simulink library "tqd"  (R2021b)
settings: Solver=VariableStepAuto  StartTime=0.0  StopTime=10.0  RelTol=1e-3
undefined symbols (not defined in the file): ATQD_AfterTqMinGain_X_Deg, ATQD_APSCreepBaseTqD_X_kph, ATQD_APSCreepBaseTqD_Y_Deg, ATQD_APSCreepBaseTqR_X_kph, ATQD_APSCreepBaseTqR_Y_Deg, ATQD_APSCreepIterm_X_kph, ATQD_APSCreepIterm_Y_kph, ATQD_APSCreepPterm_X_kph, ATQD_APSCreepPterm_Y_kph, ATQD_APSDecReq_X_kph, ATQD_APSDecReq_Y_mps2, ATQD_APSDecReqCMD_X_kph, ATQD_APSDecReqTs_X_pct, ATQD_APSDecTimeGain_X_Deg, ATQD_APSDecTimeGain_Y_s, ATQD_APSReqLowSpd_X_Deg, ATQD_AutoHoldReleaseBPS_X_Deg, ATQD_AWDLoadTrqnsGain_X_kg, ATQD_AWDLoadTrqnsGain_Y_pct, ATQD_BOSEnBPSPosn_X_kph, ATQD_BOSMap_X_rpm, ATQD_BOSMap_Y_pct, ATQD_CreepBaseTqD_X_kph, ATQD_CreepBaseTqD_Y_Deg, ATQD_CreepBaseTqR_X_kph, ATQD_CreepBaseTqR_Y_Deg, ATQD_CreepBPSDisPosn_X_Deg, ATQD_CreepBPSDisPosnR_X_Deg, ATQD_CreepBPSEnPosn_X_Deg, ATQD_CreepBPSEnPosnR_X_Deg, ATQD_CreepDeltaTq_X_kph, ATQD_CreepIterm_X_kph, ATQD_CreepIterm_Y_kph, ATQD_CreepItermMaxLimit_X_pct, ATQD_CreepPreloadTime_X_kph, ATQD_CreepPreloadTq_X_kph, ATQD_CreepPreloadTq_Y_s, ATQD_CreepProtTq_X_Deg, ATQD_CreepPterm_X_kph, ATQD_CreepPterm_Y_kph, ATQD_CreepRrTqSpRat_X_rpm, ATQD_CreepRrTqSpRat_Y_Nm, ATQD_CreepTargetSpdD_X_pct, ATQD_CreepTargetSpdR_X_pct, ATQD_ECOTqMapD_X_rpm, ATQD_ECOTqMapD_Y_pct, ATQD_EMTqMapD_X_rpm, ATQD_EMTqMapD_Y_pct, ATQD_EOPDTqMapDCon_X_rpm, ATQD_EOPDTqMapDCon_Y_Deg, ATQD_EscapeModePedTq_X_pct, ATQD_EscapeModePedTq_Y_rpm, ATQD_EscapeModePedTqFr_X_pct, ATQD_EscapeModePedTqFr_Y_rpm, ATQD_EstInitVehWeight_X_c, ATQD_FAfterTqCMDGain_X_rpm, ATQD_FAfterTqCMDGain_Y_pct, ATQD_FrLossMAPLowV_X_rpm, ATQD_FrLossMAPLowV_Y_Nm, ATQD_FrMotActReduce_X_rpm ... (+772)
libraries: simulink x211, hcu_lib x179, tqr x3
(part 10 of 28)

== system tqd/TQD/TorqueDemand/TorqueModule/OPD Hold ==
  task_time_s : Inport
  VTQD_RegenMode_enum : Inport  Port=2
  VTQD_GearActualPosn_enum : Inport  Port=3
  VTQD_VehActSpd_kph : Inport  Port=4
  VTQD_ActBPSPosn_pct : Inport  Port=5
  VVMC_ADASActive_flg : Inport  Port=6
  VVMC_CruzActive_flg : Inport  Port=7
  VTQD_ParkRequest_flg : Inport  Port=8
  VVMC_EstSlope_Deg : Inport  Port=9
  VVMC_LongAcc_Gps : Inport  Port=10
  VTQR_NoABSFEDUWhlTqReq_Nm : Inport  Port=11
  VTQR_NoABSREDUWhlTqReq_Nm : Inport  Port=12
  VINP_EPBSta_enum : Inport  Port=13
  VPMM_PwrSta_enum : Inport  Port=14
  VTQD_LowIdleAccPedal_flg : Inport  Port=15
  VTQD_ActAPSPosn_pct : Inport  Port=16
  VINP_FrPTCSActive_flg : Inport  Port=17
  VINP_RrPTCSActive_flg : Inport  Port=18
  VINP_ESCActive_flg : Inport  Port=19
  VINP_ABSActive_flg : Inport  Port=20
  VVMC_APSActive_flg : Inport  Port=21
  VTQD_PedAccTqEn_flg : Inport  Port=22
  VINP_IVICreepOnSW_flg : Inport  Port=23
  VTQD_IVIRockModeEn_flg : Inport  Port=24
  VTQD_ActWhlSkipSta_enum : Inport  Port=25
  VTQD_SkipDirect_enum : Inport  Port=26
  VTQD_LimpHomeAct_flg : Inport  Port=27
  Deceleration Calculation : Subsystem
  "OPDHold Request " : Subsystem
  Parking Requeest Backup : Subsystem
  Release Condition : Subsystem
  System Status : Subsystem
  VTQD_APSStaSys_enum : Outport
  VTQD_APSReq_enum : Outport  Port=2
  VTQD_APSDecReqA_flg : Outport  Port=3
  VTQD_APSDecReq_mps2 : Outport  Port=4
  VTQD_ActParkRequest_flg : Outport  Port=5
  VTQD_APSReqTimer_s : Outport  Port=6
  VTQD_OPDHoldEnRel_flg : Outport  Port=7
  VTQD_OPDHoldDelayForP_flg : Outport  Port=8
  VTQD_OPDHoldAllowPark_flg : Outport  Port=9
  VTQD_OPDHoldLamp_flg : Outport  Port=10
  VTQD_OPDHoldActRelTq_Nm : Outport  Port=11
  wires:
  VTQD_RegenMode_enum/1 -> [VTQD_RegenMode_enum]
  VTQD_GearActualPosn_enum/1 -> [VTQD_GearActualPosn_enum]
  VTQD_VehActSpd_kph/1 -> [VTQD_VehActSpd_kph]
  task_time_s/1 -> [task_time_s]
  [VTQD_APSStaSys_enum] -> VTQD_APSStaSys_enum/1
  [VTQD_APSReq_enum] -> VTQD_APSReq_enum/1
  [VTQD_APSDecReq_mps2] -> VTQD_APSDecReq_mps2/1
  [VTQD_APSDecReqA_flg] -> VTQD_APSDecReqA_flg/1
  VTQD_ActBPSPosn_pct/1 -> [VTQD_ActBPSPosn_pct]
  VVMC_ADASActive_flg/1 -> [VVMC_ADASActive_flg]
  VVMC_CruzActive_flg/1 -> [VVMC_CruzActive_flg]
  [VTQD_ActParkRequest_flg] -> VTQD_ActParkRequest_flg/1
  VTQD_ParkRequest_flg/1 -> [VTQD_ParkRequest_flg]
  VVMC_EstSlope_Deg/1 -> [VVMC_EstSlope_Deg]
  VVMC_LongAcc_Gps/1 -> [VVMC_LongAcc_Gps]
  VTQR_NoABSFEDUWhlTqReq_Nm/1 -> [VTQR_NoABSFEDUWhlTqReq_Nm]
  VTQR_NoABSREDUWhlTqReq_Nm/1 -> [VTQR_NoABSREDUWhlTqReq_Nm]
  VINP_EPBSta_enum/1 -> [VINP_EPBSta_enum]
  VPMM_PwrSta_enum/1 -> [VPMM_PwrSta_enum]
  [VTQD_OPDHoldDelayForP_flg] -> VTQD_OPDHoldDelayForP_flg/1
  [VTQD_APSReqTimer_s] -> VTQD_APSReqTimer_s/1
  [VTQD_OPDHoldEnRel_flg] -> VTQD_OPDHoldEnRel_flg/1
  [VTQD_AutoHoldRelease_flg] -> System Status/4(VTQD_AutiHoldRelease_flg)
  System Status/1(VTQD_APSStaSys_enum) -> [VTQD_APSStaSys_enum]
  [VTQD_ActBPSPosn_pct] -> Release Condition/5(VTQD_ActBPSPosn_pct)
  [VTQD_VehActSpd_kph] -> Release Condition/2(VTQD_VehActSpd_kph)
  Release Condition/1(VTQD_AutoHoldRelease_flg) -> [VTQD_AutoHoldRelease_flg]
  Release Condition/2(VTQD_OPDHoldEnRel_flg) -> [VTQD_OPDHoldEnRel_flg]
  System Status/2(VTQD_OPDHoldDelayForP_flg) -> [VTQD_OPDHoldDelayForP_flg]
  [VTQD_VehActSpd_kph] -> "OPDHold Request "/1(VTQD_VehActSpd_kph)
  [VTQD_APSStaSys_enum] -> "OPDHold Request "/2(VTQD_APSStaSys_enum)
  [VTQD_AutoHoldRelease_flg] -> "OPDHold Request "/3(VTQD_AutiHoldRelease_flg)
  [task_time_s] -> "OPDHold Request "/4(task_time_s)
  "OPDHold Request "/1(VTQD_APSReqTimer_s) -> [VTQD_APSReqTimer_s]
  "OPDHold Request "/2(VTQD_APSReq_enum) -> [VTQD_APSReq_enum]
  "OPDHold Request "/3(VTQD_APSDecReqA_flg) -> [VTQD_APSDecReqA_flg]
  [VTQD_VehActSpd_kph] -> Deceleration Calculation/1(VTQD_VehActSpd_kph)
  [VTQD_APSReqTimer_s] -> Deceleration Calculation/3(VTQD_APSReqTimer_s)
  [VVMC_EstSlope_Deg] -> Deceleration Calculation/4(VVMC_EstSlope_Deg)
  [VTQD_APSDecReqA_flg] -> Deceleration Calculation/5(VTQD_APSDecReqA_flg)
  Deceleration Calculation/1(VTQD_APSDecReq_mps2) -> [VTQD_APSDecReq_mps2]
  [VTQD_APSReq_enum] -> Parking Requeest Backup/1(VTQD_APSReq_enum)
  [VTQD_APSReqTimer_s] -> Parking Requeest Backup/2(VTQD_APSReqTimer_s)
  Parking Requeest Backup/1(VTQD_ActParkRequest_flg) -> [VTQD_ActParkRequest_flg]
  [VTQD_GearActualPosn_enum] -> System Status/1(VTQD_GearActualPosn_enum)
  [VINP_EPBSta_enum] -> System Status/2(VINP_EPBSta_enum)
  [VTQD_RegenMode_enum] -> System Status/3(VTQD_RegenMode_enum)
  [VVMC_ADASActive_flg] -> System Status/5(VVMC_ADASActive_flg)
  [VPMM_PwrSta_enum] -> System Status/6(VPMM_PwrSta_enum)
  [VVMC_CruzActive_flg] -> System Status/7(VVMC_CruzActive_flg)
  [VTQD_VehActSpd_kph] -> System Status/8(VTQD_VehActSpd_kph)
  [VVMC_EstSlope_Deg] -> Release Condition/1(VVMC_EstSlope_Deg)
  [VTQR_NoABSFEDUWhlTqReq_Nm] -> Release Condition/3(VTQR_NoABSFEDUWhlTqReq_Nm)
  [VTQR_NoABSREDUWhlTqReq_Nm] -> Release Condition/4(VTQR_NoABSREDUWhlTqReq_Nm)
  [task_time_s] -> Release Condition/6(task_time_s)
  [VVMC_LongAcc_Gps] -> Deceleration Calculation/2(VVMC_LongAcc_Gps)
  [VTQD_ParkRequest_flg] -> Parking Requeest Backup/3(VTQD_ParkRequest_flg)
  [VTQD_AutoHoldRelease_flg] -> Deceleration Calculation/6(VTQD_AutiHoldRelease_flg)
  [VVMC_EstSlope_Deg] -> "OPDHold Request "/5(VVMC_EstSlope_Deg)
  [VTQD_APSReqTimer_s] -> Release Condition/7(VTQD_APSReqTimer_s)
  [VTQD_LowIdleAccPedal_flg] -> Release Condition/8(VTQD_LowIdleAccPedal_flg)
  VTQD_LowIdleAccPedal_flg/1 -> [VTQD_LowIdleAccPedal_flg]
  System Status/3(VTQD_OPDHoldRgnOn2Off_flg) -> [VTQD_OPDHoldRgnOn2Off_flg]
  [VTQD_OPDHoldRgnOn2Off_flg] -> Release Condition/9(VTQD_OPDHoldRgnOn2Off_flg)
  [task_time_s] -> Parking Requeest Backup/4(task_time_s)
  [VTQD_AutoHoldRelease_flg] -> Parking Requeest Backup/5(VTQD_AutiHoldRelease_flg)
  [task_time_s] -> Deceleration Calculation/7(task_time_s)
  [VTQD_ActAPSPosn_pct] -> Deceleration Calculation/8(VTQD_ActAPSPosn_pct)
  VTQD_ActAPSPosn_pct/1 -> [VTQD_ActAPSPosn_pct]
  Parking Requeest Backup/2(VTQD_OPDHoldAllowPark_flg) -> [VTQD_OPDHoldAllowPark_flg]
  [VTQD_OPDHoldAllowPark_flg] -> VTQD_OPDHoldAllowPark_flg/1
  "OPDHold Request "/4(VTQD_OPDHoldLamp_flg) -> [VTQD_OPDHoldLamp_flg]
  [VTQD_OPDHoldLamp_flg] -> VTQD_OPDHoldLamp_flg/1
  [VTQD_OPDHoldActRelTq_Nm] -> VTQD_OPDHoldActRelTq_Nm/1
  Release Condition/3(VTQD_OPDHoldActRelTq_Nm) -> [VTQD_OPDHoldActRelTq_Nm]
  [VINP_ABSActive_flg] -> System Status/14(VINP_ABSActive_flg)
  [VVMC_EstSlope_Deg] -> System Status/9(VVMC_EstSlope_Deg)
  [task_time_s] -> System Status/10(task_time_s)
  [VINP_ESCActive_flg] -> System Status/13(VINP_ESCActive_flg)
  [VINP_FrPTCSActive_flg] -> System Status/11(VINP_FrPTCSActive_flg)
  [VINP_RrPTCSActive_flg] -> System Status/12(VINP_RrPTCSActive_flg)
  VINP_FrPTCSActive_flg/1 -> [VINP_FrPTCSActive_flg]
  VINP_RrPTCSActive_flg/1 -> [VINP_RrPTCSActive_flg]
  VINP_ESCActive_flg/1 -> [VINP_ESCActive_flg]
  VINP_ABSActive_flg/1 -> [VINP_ABSActive_flg]
  [VVMC_APSActive_flg] -> System Status/15(VVMC_APSActive_flg)
  VVMC_APSActive_flg/1 -> [VVMC_APSActive_flg]
  VTQD_PedAccTqEn_flg/1 -> [VTQD_PedAccTqEn_flg]
  VINP_IVICreepOnSW_flg/1 -> [VINP_IVICreepOnSW_flg]
  [VTQD_PedAccTqEn_flg] -> System Status/16(VTQD_PedAccTqEn_flg)
  [VINP_IVICreepOnSW_flg] -> System Status/17(VINP_IVICreepOnSW_flg)
  [VTQD_IVIRockModeEn_flg] -> System Status/18(VTQD_IVIRockModeEn_flg)
  VTQD_IVIRockModeEn_flg/1 -> [VTQD_IVIRockModeEn_flg]
  VTQD_SkipDirect_enum/1 -> [VTQD_SkipDirect_enum]
  VTQD_ActWhlSkipSta_enum/1 -> [VTQD_ActWhlSkipSta_enum]
  [VTQD_ActWhlSkipSta_enum] -> System Status/19(VTQD_ActWhlSkipSta_enum)
  [VTQD_SkipDirect_enum] -> System Status/20(VTQD_SkipDirect_enum)
  [VTQD_LimpHomeAct_flg] -> System Status/21(VTQD_LimpHomeAct_flg)
  VTQD_LimpHomeAct_flg/1 -> [VTQD_LimpHomeAct_flg]

== system tqd/TQD/TorqueDemand/TorqueModule/Signal for ESC ==
  note: Front/Raer EDU actual torque (After Gearbox) calculation
  note: Front/Rear MCU error status signals
  note: Driving torque reduction permission status
  note: Front/Rear EDU speed (After Gearbox) calculation
  note: Front/Rear EDU rolling regen torque calculation
  VINP_FrEDURealTMTq_Nm : Inport
  VINP_RrEDURealTMTq_Nm : Inport  Port=2
  VTQD_RollRegenEnable_flg : Inport  Port=3
  VINP_FrntAxlTrqReqBrk_Nm : Inport  Port=4
  VINP_RearAxlTrqReqBrk_Nm : Inport  Port=5
  VINP_FrTMSpd_rpm : Inport  Port=6
  VINP_RrTMSpd_rpm : Inport  Port=7
  VINP_FrRBCActive_flg : Inport  Port=8
  VINP_RrRBCActive_flg : Inport  Port=9
  VTQR_ActualFEDUWhlTqReq_Nm : Inport  Port=10
  VTQR_ActualREDUWhlTqReq_Nm : Inport  Port=11
  VTQR_NoABSFEDUWhlTqReq_Nm : Inport  Port=12
  VTQR_NoABSREDUWhlTqReq_Nm : Inport  Port=13
  VTQD_DriverWhlTqDem_Nm : Inport  Port=14
  VVMC_ADASActive_flg : Inport  Port=15
  VVMC_ACCRequiredAccel_mps2 : Inport  Port=16
  VINP_HVBattSOC_pct : Inport  Port=17
  VTQD_AfterAvailableTqDemFr_Nm : Inport  Port=18
  VTQD_AfterAvailableTqDemRr_Nm : Inport  Port=19
  VTQD_GearActualPosn_enum : Inport  Port=20
  VPMM_DrivetrainSelect_enum : Inport  Port=21
  VDDM_RegenErrCFS_flg : Inport  Port=22
  AND1 : Logic  AllPortsSameDT=off  OutDataTypeStr=boolean
  AND2 : Logic  AllPortsSameDT=off  OutDataTypeStr=boolean
  Abs{,1..3} (4 alike) : Abs
  Constant1 : Constant  Value=KTQD_AvailBRgnTqVSOC_pct
  Constant{7,10,23,25,45,47..48,50} (8 alike) : Constant  Value=ZERO_FLOAT
  Constant{3,5,8,11,34,42} (6 alike) : Constant  Value=FALSE
  Constant{2,4,9,12,29,40} (6 alike) : Constant  Value=TRUE
  Constant13 : Constant  Value=KTQD_BRegenCalEnTq_Nm
  Constant{14,16,18,20} (4 alike) : Constant  Value=eps
  Constant15 : Constant  Value=KTQD_AvailBRgnTqVSOC_pct
  Constant{17,19,21..22,24,26,44,52} (8 alike) : Constant  Value=ONE_FLOAT
  Constant27 : Constant  Value=KTQD_FrAvailBRgnTqV_flg_ovrdflg
  Constant28 : Constant  Value=KTQD_FrAvailBRgnTqV_flg_ovrdval
  Constant30 : Constant  Value=KTQD_RrAvailBRgnTqV_flg_ovrdflg
  Constant31 : Constant  Value=KTQD_RrAvailBRgnTqV_flg_ovrdval
  Constant32 : Constant  Value=KTQD_DecideEDUActTqSW_flg
  Constant33 : Constant  Value=KTQD_DecideEDUActTqSW_flg
  Constant35 : Constant  Value=ENUM_DRIVETRAIN_AWD
  Constant36 : Constant  Value=ENUM_DRIVETRAIN_FWD
  Constant37 : Constant  Value=ENUM_DRIVETRAIN_AWD
  Constant38 : Constant  Value=ENUM_DRIVETRAIN_RWD
  Constant39 : Constant  Value=KTQD_BRegenCalEnTq_Nm
  Constant41 : Constant  Value=ENUM_GEARACTUALPOSN_R
  Constant43 : Constant  Value=KVMC_ACCReqCMdBond_mps2
  Constant46 : Constant  Value=MINUSONE_FLOAT
  Constant49 : Constant  Value=KVMC_ACCReqCMdBond_mps2
  Constant51 : Constant  Value=ENUM_GEARACTUALPOSN_R
  Constant53 : Constant  Value=MINUSONE_FLOAT
  Constant6 : Constant  Value=KTQD_PTCSPermSta_flg
  Data Type Conversion{1..3,5..7} (6 alike) : DataTypeConversion  OutDataTypeStr=single
  Delay{,1..3} (4 alike) : Delay  DelayLength=1
  Divide{,1,3,5} (4 alike) : Product  Inputs=*/
  Divide{2,4,6..7} (4 alike) : Product  Inputs=**
  Equal{,1..3,8..9} (6 alike) : RelationalOperator  Operator=<  OutDataTypeStr=boolean  RndMeth=Simplest
  Equal{4..7,10..11} (6 alike) : RelationalOperator  Operator===  OutDataTypeStr=boolean  RndMeth=Simplest
  Gain1 : Gain  Gain=1/KTQD_FrTMTotalGearRatio_gain
  Gain{4,6..7,10} (4 alike) : Gain  Gain=KTQD_RrTMTotalGearRatio_gain
  Gain2 : Gain  Gain=1/KTQD_RrTMTotalGearRatio_gain
  Gain{3,5,8..9} (4 alike) : Gain  Gain=KTQD_FrTMTotalGearRatio_gain
  Logical Operator : Logic  Operator=OR  AllPortsSameDT=off  OutDataTypeStr=boolean
  Logical Operator1 : Logic  AllPortsSameDT=off  OutDataTypeStr=boolean
  Logical Operator2 : Logic  AllPortsSameDT=off  OutDataTypeStr=boolean
  Max : MinMax  Function=max  Inputs=2
  Max1 : MinMax  Function=max  Inputs=2
  OR{,1..7} (8 alike) : Logic  Operator=OR  AllPortsSameDT=off  OutDataTypeStr=boolean
  Product : Product
  Product1 : Product
  Relational Operator{,1,4..5} (4 alike) : RelationalOperator  Operator=<=  OutDataTypeStr=boolean  RndMeth=Simplest
  Relational Operator2 : RelationalOperator  Operator=<  OutDataTypeStr=boolean  RndMeth=Simplest
  Relational Operator3 : RelationalOperator  Operator=<  OutDataTypeStr=boolean  RndMeth=Simplest
  Relational Operator6 : RelationalOperator  OutDataTypeStr=boolean  RndMeth=Simplest
  Relational Operator7 : RelationalOperator  OutDataTypeStr=boolean  RndMeth=Simplest
  Saturation : Saturate  UpperLimit=KTQD_FrBRgnCalUpLim_Nm  LowerLimit=KTQD_FrBRgnCalLowLim_Nm
      settings: AttributesFormatString=|
      | UpperLimit: %<UpperLimit>
      | LowerLimit: %<LowerLimit>
  Saturation1 : Saturate  UpperLimit=KTQD_RrBRgnCalUpLim_Nm  LowerLimit=KTQD_RrBRgnCalLowLim_Nm
      settings: AttributesFormatString=|
      | UpperLimit: %<UpperLimit>
      | LowerLimit: %<LowerLimit>
  Saturation2 : Saturate  UpperLimit=KTQD_RrEDURollRgnUpTq_Nm  LowerLimit=KTQD_RrEDURollRgnLowTq_Nm
      settings: AttributesFormatString=|
      | UpperLimit: %<UpperLimit>
      | LowerLimit: %<LowerLimit>
  Saturation3 : Saturate  UpperLimit=KTQD_FrEDURollRgnUpTq_Nm  LowerLimit=KTQD_FrEDURollRgnLowTq_Nm
  Saturation{4..7} (4 alike) : Saturate  UpperLimit=KTQD_TMTqDeviationUp_c  LowerLimit=KTQD_TMTqDeviationLow_c
      Saturation4 settings: AttributesFormatString=|
      | UpperLimit: %<UpperLimit>
      | LowerLimit: %<LowerLimit>
      Saturation5 settings: AttributesFormatString=|
      | UpperLimit: %<UpperLimit>
      | LowerLimit: %<LowerLimit>
      Saturation6 settings: LockScale=on
      Saturation6 settings: AttributesFormatString=|
      | UpperLimit: %<UpperLimit>
      | LowerLimit: %<LowerLimit>
      Saturation7 settings: AttributesFormatString=|
      | UpperLimit: %<UpperLimit>
      | LowerLimit: %<LowerLimit>
  Switch{,1..18,20..21,23} (22 alike) : Switch  Criteria=u2 ~= 0
  Switch{19,22,24..27} (6 alike) : Switch  Criteria=u2 > Threshold
  VTQD_FrEDUActTq_Nm : Outport
  VTQD_RrEDUActTq_Nm : Outport  Port=2
  VTQD_FrEDURolRgnTq_Nm : Outport  Port=3
  VTQD_RrEDURolRgnTq_Nm : Outport  Port=4
  VTQD_FrEDUSpd_rpm : Outport  Port=5
  VTQD_RrEDUSpd_rpm : Outport  Port=6
  VTQD_FrEDUSpdValid_flg : Outport  Port=7
  VTQD_FrEDUActTqValid_flg : Outport  Port=8
  VTQD_FrEDURolRgnTqValid_flg : Outport  Port=9
  VTQD_FrEDUAvailBrkRgnTqV_flg : Outport  Port=10
  VTQD_RrEDUSpdValid_flg : Outport  Port=11
  VTQD_RrEDUActTqValid_flg : Outport  Port=12
  VTQD_RrEDURolRgnTqValid_flg : Outport  Port=13
  VTQD_RrEDUAvailBrkRgnTqV_flg : Outport  Port=14
  VTQD_RgnAbnorSta_flg : Outport  Port=15
  VTQD_PTCSPermSta_flg : Outport  Port=16
  wires:
  Gain2/1 -> Data Type Conversion6/1
  Logical Operator/1 -> VTQD_RgnAbnorSta_flg/1  "VTQD_RgnAbnorSta_flg"
  Switch3/1 -> Logical Operator/1, VTQD_FrEDURolRgnTqValid_flg/1, VTQD_FrEDUActTqValid_flg/1, VTQD_FrEDUSpdValid_flg/1
  [VINP_FrTMSpd_rpm] -> Gain1/1
  Data Type Conversion2/1 -> VTQD_FrEDURolRgnTq_Nm/1  "VTQD_FrEDURolRgnTq_Nm"
  Data Type Conversion5/1 -> VTQD_FrEDUSpd_rpm/1  "VTQD_FrEDUSpd_rpm"
  Data Type Conversion3/1 -> VTQD_RrEDURolRgnTq_Nm/1  "VTQD_RrEDURolRgnTq_Nm"
  [VINP_RrTMSpd_rpm] -> Gain2/1
  Data Type Conversion6/1 -> VTQD_RrEDUSpd_rpm/1  "VTQD_RrEDUSpd_rpm"
  Switch2/1 -> VTQD_RrEDUActTqValid_flg/1, Logical Operator/2, VTQD_RrEDUSpdValid_flg/1, VTQD_RrEDURolRgnTqValid_flg/1
  Gain1/1 -> Data Type Conversion5/1
  Constant25/1 -> Relational Operator3/2
  [VINP_FrEDURealTMTq_Nm] -> Gain8/1
  Equal/1 -> Switch12/2
  [VINP_RrEDURealTMTq_Nm] -> Gain7/1
  Switch12/1 -> Switch14/3, Relational Operator2/1  "VTQD_FrTMTqDeviation_c"
  Constant21/1 -> Switch12/1
  [VTQR_ActualREDUWhlTqReq_Nm] -> Delay1/1
  Gain3/1 -> Divide/1
  Gain7/1 -> Saturation1/1
  Constant23/1 -> Relational Operator2/2
  [VINP_RrEDURealTMTq_Nm] -> Gain4/1
  Divide3/1 -> Switch13/3
  Divide/1 -> Switch12/3
  Delay/1 -> Divide/2, Abs2/1
  [VINP_FrEDURealTMTq_Nm] -> Gain3/1
  Switch15/1 -> Saturation5/1  "VTQD_ActRrTMTqDeviation_c"
  [VTQR_ActualFEDUWhlTqReq_Nm] -> Delay/1
  Relational Operator2/1 -> Switch14/2
  Constant26/1 -> Switch15/1
  Switch13/1 -> Switch15/3, Relational Operator3/1  "VTQD_RrTMTqDeviation_c"
  Constant22/1 -> Switch13/1
  Saturation4/1 -> Divide2/2
  Gain8/1 -> Saturation/1
  Gain4/1 -> Divide3/1
  Relational Operator3/1 -> Switch15/2
  Constant24/1 -> Switch14/1
  Switch14/1 -> Saturation4/1  "VTQD_ActFrTMTqDeviation_c"
  Divide2/1 -> Data Type Conversion1/1  "VTQD_FrBRegenCal_Nm"
  Saturation5/1 -> Divide4/2
  Divide4/1 -> Data Type Conversion7/1  "VTQD_RrBRegenCal_Nm"
  Delay1/1 -> Abs3/1, Divide3/2
  Equal2/1 -> Switch13/2
  Gain5/1 -> Divide1/1
  Switch8/1 -> Divide1/2
  OR/1 -> Switch4/2
  Switch5/1 -> OR/2  "VTQD_FrWhlTqDemNeg_flg"
  Delay2/1 -> Abs/1, Switch8/3
  [VTQR_ActualFEDUWhlTqReq_Nm] -> Delay2/1
  Constant17/1 -> Switch8/1
  [VTQD_DriverWhlTqDem_Nm] -> Relational Operator/1
  Constant9/1 -> Switch5/1
  Equal1/1 -> Switch8/2
  [VTQD_RollRegenEnable_flg] -> OR/1
  [VINP_FrEDURealTMTq_Nm] -> Gain5/1
  Switch4/1 -> Saturation3/1
  Constant7/1 -> Relational Operator/2
  Divide6/1 -> Switch4/1  "VTQD_FrARegenCal_Nm"
  [VTQR_NoABSFEDUWhlTqReq_Nm] -> Divide6/1
  Relational Operator/1 -> Switch5/2
  Constant8/1 -> Switch5/3
  Saturation3/1 -> Data Type Conversion2/1
  Saturation6/1 -> Divide6/2  "VTQD_FrARgnTqDeviation_c"
  Divide1/1 -> Saturation6/1
  Constant10/1 -> Relational Operator1/2
  Gain6/1 -> Divide5/1
  Delay3/1 -> Abs1/1, Switch11/3
  [VTQR_ActualREDUWhlTqReq_Nm] -> Delay3/1
  Switch6/1 -> Saturation2/1
  Saturation2/1 -> Data Type Conversion3/1
  OR1/1 -> Switch6/2
  [VINP_RrEDURealTMTq_Nm] -> Gain6/1
  [VTQD_RollRegenEnable_flg] -> OR1/1
  Constant12/1 -> Switch9/1
  Switch9/1 -> OR1/2  "VTQD_RrWhlTqDemNeg_flg"
  [VTQD_DriverWhlTqDem_Nm] -> Relational Operator1/1
  [VTQR_NoABSREDUWhlTqReq_Nm] -> Divide7/1
  Equal3/1 -> Switch11/2
  Saturation7/1 -> Divide7/2  "VTQD_RrARgnTqDeviation_c"
  Divide7/1 -> Switch6/1  "VTQD_RrARegenCal_Nm"
  Switch11/1 -> Divide5/2
  Constant19/1 -> Switch11/1
  Divide5/1 -> Saturation7/1
  Constant11/1 -> Switch9/3
  Relational Operator1/1 -> Switch9/2
  Constant30/1 -> Switch17/2
  Constant31/1 -> Switch17/1
  Constant28/1 -> Switch16/1
  Constant27/1 -> Switch16/2
  Switch16/1 -> VTQD_FrEDUAvailBrkRgnTqV_flg/1
  Switch17/1 -> VTQD_RrEDUAvailBrkRgnTqV_flg/1
  Constant2/1 -> Switch2/1
  Logical Operator1/1 -> Switch3/2
  Constant5/1 -> Switch3/3
  Constant4/1 -> Switch3/1
  Constant3/1 -> Switch2/3
  VINP_FrEDURealTMTq_Nm/1 -> [VINP_FrEDURealTMTq_Nm]
  VINP_RrEDURealTMTq_Nm/1 -> [VINP_RrEDURealTMTq_Nm]
  VTQD_RollRegenEnable_flg/1 -> [VTQD_RollRegenEnable_flg]
  VINP_FrntAxlTrqReqBrk_Nm/1 -> [VINP_FrntAxlTrqReqBrk_Nm]
  VTQR_ActualFEDUWhlTqReq_Nm/1 -> [VTQR_ActualFEDUWhlTqReq_Nm]
  VTQR_ActualREDUWhlTqReq_Nm/1 -> [VTQR_ActualREDUWhlTqReq_Nm]
  VTQR_NoABSFEDUWhlTqReq_Nm/1 -> [VTQR_NoABSFEDUWhlTqReq_Nm]
  VTQR_NoABSREDUWhlTqReq_Nm/1 -> [VTQR_NoABSREDUWhlTqReq_Nm]
  VTQD_DriverWhlTqDem_Nm/1 -> [VTQD_DriverWhlTqDem_Nm]
  VINP_FrRBCActive_flg/1 -> [VINP_FrRBCActive_flg]
  VINP_FrTMSpd_rpm/1 -> [VINP_FrTMSpd_rpm]
  VINP_RrTMSpd_rpm/1 -> [VINP_RrTMSpd_rpm]
  VINP_RearAxlTrqReqBrk_Nm/1 -> [VINP_RearAxlTrqReqBrk_Nm]
  VINP_RrRBCActive_flg/1 -> [VINP_RrRBCActive_flg]
  AND1/1 -> Switch10/2
  Constant13/1 -> Relational Operator4/2
  [VINP_FrRBCActive_flg] -> AND2/1
  AND2/1 -> Switch7/2
  Constant39/1 -> Relational Operator5/2
  [VINP_RrRBCActive_flg] -> AND1/1
  Data Type Conversion1/1 -> Switch1/3
  Switch1/1 -> Switch7/1
  VVMC_ADASActive_flg/1 -> [VVMC_ADASActive_flg]
  [VVMC_ADASActive_flg] -> Switch1/2
  [VINP_FrntAxlTrqReqBrk_Nm] -> Switch1/1
  Data Type Conversion7/1 -> Switch18/3
  Switch18/1 -> Switch10/1
  [VINP_RearAxlTrqReqBrk_Nm] -> Switch18/1
  Constant34/1 -> Switch20/1
  Constant40/1 -> Switch21/3
  Constant29/1 -> Switch20/3
  Constant42/1 -> Switch21/1
  Switch21/1 -> Switch17/3
  Switch20/1 -> Switch16/3
  OR5/1 -> AND2/2
  OR4/1 -> AND1/2
  [VTQR_NoABSFEDUWhlTqReq_Nm] -> Switch19/3
  Constant47/1 -> Switch19/1
  Switch19/1 -> Switch4/3
  [VVMC_ADASActive_flg] -> Switch19/2
  Switch22/1 -> Switch6/3
  Constant45/1 -> Switch22/1
  [VTQR_NoABSREDUWhlTqReq_Nm] -> Switch22/3
  [VVMC_ADASActive_flg] -> Switch22/2
  Saturation/1 -> Switch/3
  Constant43/1 -> Equal8/2
  Equal8/1 -> Switch/2
  VVMC_ACCRequiredAccel_mps2/1 -> [VVMC_ACCRequiredAccel_mps2]
  [VVMC_ACCRequiredAccel_mps2] -> Equal8/1
  Switch/1 -> Switch7/3
  Constant48/1 -> Switch/1
  Constant50/1 -> Switch23/1
  Equal9/1 -> Switch23/2
  [VVMC_ACCRequiredAccel_mps2] -> Equal9/1
  Constant49/1 -> Equal9/2
  Saturation1/1 -> Switch23/3
  Switch23/1 -> Switch10/3
  Constant14/1 -> Equal/2
  Constant16/1 -> Equal2/2
  Constant18/1 -> Equal1/2
  Constant20/1 -> Equal3/2
  [VVMC_ADASActive_flg] -> Switch18/2
  [VINP_HVBattSOC_pct] -> Relational Operator6/1
  Constant1/1 -> Relational Operator6/2
  OR6/1 -> Switch21/2
  Relational Operator6/1 -> OR6/1
  [VVMC_ADASActive_flg] -> OR6/2
  Constant15/1 -> Relational Operator7/2
  Relational Operator7/1 -> OR7/1
  [VINP_HVBattSOC_pct] -> Relational Operator7/1
  OR7/1 -> Switch20/2
  [VVMC_ADASActive_flg] -> OR7/2
  VINP_HVBattSOC_pct/1 -> [VINP_HVBattSOC_pct]
  Abs/1 -> Equal1/1
  Abs1/1 -> Equal3/1
  Abs2/1 -> Equal/1
  Abs3/1 -> Equal2/1
  VTQD_AfterAvailableTqDemFr_Nm/1 -> [VTQD_AfterAvailableTqDemFr_Nm]
  VTQD_AfterAvailableTqDemRr_Nm/1 -> [VTQD_AfterAvailableTqDemRr_Nm]
  Constant6/1 -> VTQD_PTCSPermSta_flg/1  "VTQD_PTCSPermSta_flg"
  [VVMC_ADASActive_flg] -> OR5/1
  [VTQR_NoABSFEDUWhlTqReq_Nm] -> Switch24/3
  Switch24/1 -> Relational Operator4/1
  Relational Operator4/1 -> OR5/2
  Constant32/1 -> Switch24/2
  [VTQD_AfterAvailableTqDemFr_Nm] -> Switch24/1
  Constant33/1 -> Switch25/2
  [VTQD_AfterAvailableTqDemRr_Nm] -> Switch25/1
  Switch25/1 -> Relational Operator5/1
  [VTQR_NoABSREDUWhlTqReq_Nm] -> Switch25/3
  [VVMC_ADASActive_flg] -> OR4/1
  Relational Operator5/1 -> OR4/2
  VTQD_GearActualPosn_enum/1 -> [VTQD_GearActualPosn_enum]
  Switch7/1 -> Product/2
  Product/1 -> VTQD_FrEDUActTq_Nm/1  "VTQD_FrEDUActTq_Nm"
  Equal10/1 -> Switch26/2
  [VTQD_GearActualPosn_enum] -> Equal10/1
  Switch26/1 -> Product/1
  Constant41/1 -> Equal10/2
  Constant44/1 -> Switch26/3
  Constant46/1 -> Switch26/1
  Equal11/1 -> Switch27/2
  [VTQD_GearActualPosn_enum] -> Equal11/1
  Constant51/1 -> Equal11/2
  Constant53/1 -> Switch27/1
  Switch27/1 -> Product1/1
  Constant52/1 -> Switch27/3
  Switch10/1 -> Product1/2
  Product1/1 -> VTQD_RrEDUActTq_Nm/1  "VTQD_RrEDUActTq_Nm"
  [VINP_FrntAxlTrqReqBrk_Nm] -> Max/2
  Max/1 -> Divide2/1
  [VINP_FrEDURealTMTq_Nm] -> Gain9/1
  Gain9/1 -> Max/1
  Gain10/1 -> Max1/1
  [VINP_RearAxlTrqReqBrk_Nm] -> Max1/2
  [VINP_RrEDURealTMTq_Nm] -> Gain10/1
  Max1/1 -> Divide4/1
  VDDM_RegenErrCFS_flg/1 -> [VDDM_RegenErrCFS_flg]
  VPMM_DrivetrainSelect_enum/1 -> [VPMM_DrivetrainSelect_enum]
  [VDDM_RegenErrCFS_flg] -> Logical Operator1/2
  OR2/1 -> Logical Operator1/1
  [VPMM_DrivetrainSelect_enum] -> Equal5/1
  Constant35/1 -> Equal4/2
  Constant36/1 -> Equal5/2
  Equal4/1 -> OR2/1
  Equal5/1 -> OR2/2
  [VPMM_DrivetrainSelect_enum] -> Equal4/1
  Constant37/1 -> Equal6/2
  Equal7/1 -> OR3/2
  Constant38/1 -> Equal7/2
  [VPMM_DrivetrainSelect_enum] -> Equal7/1
  OR3/1 -> Logical Operator2/1
  [VDDM_RegenErrCFS_flg] -> Logical Operator2/2
  Equal6/1 -> OR3/1
  Logical Operator2/1 -> Switch2/2
  [VPMM_DrivetrainSelect_enum] -> Equal6/1

== system tqd/TQD/TorqueDemand/TorqueModule/Signals for BCM ==
  VTQD_ARegenActive_flg : Inport
  VINP_LongAccel_Gps : Inport  Port=2
  Constant : Constant  Value=KVMC_GravityValue_mps2
  Logical Operator : Logic  AllPortsSameDT=off  OutDataTypeStr=boolean
  Product : Product
  Relay1 : Relay  OnSwitchValue=KTQD_RegBrkLPOff_c  OffSwitchValue=KTQD_RegBrkLPOn_c  OnOutputValue=0  OffOutputValue=1
      settings: AttributesFormatString=|
      | ON: %<OnSwitchValue>
      | OFF: %<OffSwitchValue>
  VTQD_ReBrakeLPReq_flg : Outport
  wires:
  VINP_LongAccel_Gps/1 -> [VINP_LongAccel_Gps]
  Relay1/1 -> Logical Operator/2
  Logical Operator/1 -> VTQD_ReBrakeLPReq_flg/1  "VTQD_ReBrakeLPReq_flg"
  Constant/1 -> Product/1
  [VTQD_ARegenActive_flg] -> Logical Operator/1
  Product/1 -> Relay1/1
  [VINP_LongAccel_Gps] -> Product/2
  VTQD_ARegenActive_flg/1 -> [VTQD_ARegenActive_flg]

== system tqd/TQD/TorqueDemand/TorqueModule/Signals for MCU ==
  Constant : Constant  Value=KTQD_FrIdcMin_A
  Constant1 : Constant  Value=KTQD_FrIdcMax_A
  Constant2 : Constant  Value=KTQD_FrUdcMax_V
  Constant3 : Constant  Value=KTQD_FrUdcMin_V
  Constant4 : Constant  Value=KTQD_RrIdcMin_A
  Constant5 : Constant  Value=KTQD_RrIdcMax_A
  Constant6 : Constant  Value=KTQD_RrUdcMax_V
  Constant7 : Constant  Value=KTQD_RrUdcMin_V
  VTQD_FrIdcMin_A : Outport
  VTQD_FrIdcMax_A : Outport  Port=2
  VTQD_FrUdcMin_V : Outport  Port=3
  VTQD_FrUdcMax_V : Outport  Port=4
  VTQD_RrIdcMin_A : Outport  Port=5
  VTQD_RrIdcMax_A : Outport  Port=6
  VTQD_RrUdcMin_V : Outport  Port=7
  VTQD_RrUdcMax_V : Outport  Port=8
  wires:
  Constant4/1 -> VTQD_RrIdcMin_A/1  "VTQD_RrIdcMin_A"
  Constant6/1 -> VTQD_RrUdcMax_V/1  "VTQD_RrUdcMax_V"
  Constant5/1 -> VTQD_RrIdcMax_A/1  "VTQD_RrIdcMax_A"
  Constant7/1 -> VTQD_RrUdcMin_V/1  "VTQD_RrUdcMin_V"
  Constant2/1 -> VTQD_FrUdcMax_V/1  "VTQD_FrUdcMax_V"
  Constant3/1 -> VTQD_FrUdcMin_V/1  "VTQD_FrUdcMin_V"
  Constant1/1 -> VTQD_FrIdcMax_A/1  "VTQD_FrIdcMax_A"
  Constant/1 -> VTQD_FrIdcMin_A/1  "VTQD_FrIdcMin_A"

== system tqd/TQD/TorqueDemand/TorqueModule/TqCoordination ==
  note: Wheel torque coordination
  VTQD_GearActualPosn_enum : Inport
  VVMC_ADASActive_flg : Inport  Port=2
  VVMC_ADASWhlTqReq_Nm : Inport  Port=3
  VVMC_CruzActive_flg : Inport  Port=4
  VVMC_CruzWhlTqReq_Nm : Inport  Port=5
  VVMC_MSAActive_flg : Inport  Port=6
  VVMC_MSAWhlTqReq_Nm : Inport  Port=7
  VVMC_APSActive_flg : Inport  Port=8
  VTQD_DriverWhlTqDem_Nm : Inport  Port=9
  VINP_ADASForceIdle_flg : Inport  Port=10
  VTQD_PreLoadHold_flg : Inport  Port=11
  VINP_HVBPwrAvailDchrg_kW : Inport  Port=12
  VINP_HVBPwrAvailChrg_kW : Inport  Port=13
  VTQD_MotorLossTotal_kw : Inport  Port=14
  VTQD_FrShaftSpd_rpm : Inport  Port=15
  VTQD_RrShaftSpd_rpm : Inport  Port=16
  Constant1 : Constant  Value=ENUM_GEARACTUALPOSN_R
  Constant2 : Constant  Value=ENUM_GEARACTUALPOSN_D
  Constant3 : Constant  Value=KTQD_NewTotalCapTqSW_flg
  Coordinate_ADAS : Subsystem  AncestorBlock=tqd162/TQD/TorqueDemand/TorqueModule/TqCoordination/Coordinate_FrADAS  TreatAsAtomicUnit=on
  Coordinate_ADASForceIdle : Subsystem  TreatAsAtomicUnit=on
  Coordinate_APS : Subsystem  TreatAsAtomicUnit=on
  Coordinate_Cruise : Subsystem  AncestorBlock=tqd162/TQD/TorqueDemand/TorqueModule/TqCoordination/Coordinate_FrCruise  TreatAsAtomicUnit=on
  Coordinate_DirverPedal : Subsystem  AncestorBlock=tqd/TQD/TorqueDemand/TorqueModule/TqCoordination/If Action Subsystem4  TreatAsAtomicUnit=on
  Coordinate_MSA : Subsystem  AncestorBlock=tqd162/TQD/TorqueDemand/TorqueModule/TqCoordination/Coordinate_FrMSA  TreatAsAtomicUnit=on
  Coordinate_NoSuitbleGear_flg : Subsystem  TreatAsAtomicUnit=on
  Data Type Conversion2 : DataTypeConversion  OutDataTypeStr=uint8
  Equal1 : RelationalOperator  Operator===  OutDataTypeStr=boolean  RndMeth=Simplest
  Equal4 : RelationalOperator  Operator===  OutDataTypeStr=boolean  RndMeth=Simplest
  If : If  NumInputs=6  IfExpression=u1 ~= 0  ElseIfExpressions=u2 ~= 0, u3 ~= 0, u4 ~= 0, u5 ~= 0, u6 ~= 0
  Merge4 : Merge  Inputs=7
  Merge5 : Merge  Inputs=7
  NOT1 : Logic  Operator=NOT  AllPortsSameDT=off  OutDataTypeStr=boolean
  OR1 : Logic  Operator=OR  AllPortsSameDT=off  OutDataTypeStr=boolean
  Saturation Dynamic : simulink/Discontinuities/Saturation Dynamic  OutMin=[]  OutMax=[]  OutDataTypeStr=Inherit: Same as second input  OutDataType=fixdt(1, 16)  OutScaling=2^-10  DoSatur=off
  Switch : Switch  Criteria=u2 ~= 0
      settings: AttributesFormatString=%<Criteria>
  "Total Demand Capacity Torque " : Subsystem
  VTQD_CoordTqDem_Nm : Outport
  VTQD_TqSource_enum : Outport  Port=2
  wires:
  Coordinate_ADASForceIdle/2(VTQD_ADASForceIdle_enum) -> [VTQD_ADASForceIdle_enum]
  Coordinate_ADASForceIdle/1(VTQD_ADASForceIdleReq_Nm) -> [VTQD_ADASForceIdleReq_Nm]
  Coordinate_DirverPedal/2(VTQD_TqSourceInternal_enum) -> [VTQD_TqSourceInternal_enum]
  Coordinate_DirverPedal/1(VTQD_DriverWhlTqReq_Nm) -> [VTQD_DriverWhlTqReq_Nm]
  [VTQD_NoSuitbleGear_flg] -> If/1
  Equal4/1 -> OR1/1
  Constant2/1 -> Equal4/1
  VTQD_GearActualPosn_enum/1 -> [VTQD_GearActualPosn_enum]
  Coordinate_NoSuitbleGear_flg/1(VTQD_GearNoSuitReq_Nm) -> [VTQD_GearNoSuitReq_Nm]
  OR1/1 -> NOT1/1
  Coordinate_APS/1(VTQD_APSWhlTqReq_Nm) -> [VTQD_APSWhlTqReq_Nm]
  Coordinate_APS/2(VTQD_TqSourceAPS_enum) -> [VTQD_TqSourceAPS_enum]
  NOT1/1 -> [VTQD_NoSuitbleGear_flg]  "VTQD_NoSuitbleGear_flg"
  [VTQD_GearActualPosn_enum] -> Equal4/2, Equal1/1
  Equal1/1 -> OR1/2
  Coordinate_NoSuitbleGear_flg/2(VTQD_TqSourceGearNoSuit_enum) -> [VTQD_TqSourceGearNoSuit_enum]
  Constant1/1 -> Equal1/2
  VVMC_ADASActive_flg/1 -> [VVMC_ADASActive_flg]
  VTQD_DriverWhlTqDem_Nm/1 -> [VTQD_DriverWhlTqDem_Nm]
  VVMC_ADASWhlTqReq_Nm/1 -> [VVMC_ADASWhlTqReq_Nm]
  VINP_ADASForceIdle_flg/1 -> [VINP_ADASForceIdle_flg]
  VVMC_MSAActive_flg/1 -> [VVMC_MSAActive_flg]
  VVMC_CruzWhlTqReq_Nm/1 -> [VVMC_CruzWhlTqReq_Nm]
  VVMC_MSAWhlTqReq_Nm/1 -> [VVMC_MSAWhlTqReq_Nm]
  VVMC_APSActive_flg/1 -> [VVMC_APSActive_flg]
  VVMC_CruzActive_flg/1 -> [VVMC_CruzActive_flg]
  VTQD_PreLoadHold_flg/1 -> [VTQD_PreLoadHold_flg]
  If/1 -> Coordinate_NoSuitbleGear_flg/Action
  Coordinate_ADAS/1(VTQD_ADASWhlTqReq_Nm) -> [VTQD_ADASWhlTqReq_Nm]
  Coordinate_ADAS/2(VTQD_TqSourceADAS_enum) -> [VTQD_TqSourceADAS_enum]
  [VTQD_PreLoadHold_flg] -> Coordinate_ADAS/2(VTQD_PreLoadHold_flg)
  Coordinate_Cruise/2(VTQD_TqSourceCruz_enum) -> [VTQD_TqSourceCruz_enum]
  Coordinate_MSA/2(VTQD_TqSourceMSA_enum) -> [VTQD_TqSourceMSA_enum]
  Coordinate_Cruise/1(VTQD_CruzWhlTqReq_Nm) -> [VTQD_CruzWhlTqReq_Nm]
  Coordinate_MSA/1(VTQD_MSAWhlTqReq_Nm) -> [VTQD_MSAWhlTqReq_Nm]
  [VINP_ADASForceIdle_flg] -> If/2
  [VVMC_ADASActive_flg] -> If/3
  [VVMC_CruzActive_flg] -> If/4
  [VVMC_MSAActive_flg] -> If/5
  [VVMC_APSActive_flg] -> If/6
  If/2 -> Coordinate_ADASForceIdle/Action
  If/3 -> Coordinate_ADAS/Action
  [VVMC_ADASWhlTqReq_Nm] -> Coordinate_ADAS/1(VVMC_ADASWhlTqReq_Nm)
  [VTQD_DriverWhlTqDem_Nm] -> Coordinate_ADAS/3(VTQD_DriverWhlTqDem_Nm)
  If/4 -> Coordinate_Cruise/Action
  [VVMC_CruzWhlTqReq_Nm] -> Coordinate_Cruise/1(VVMC_CruzWhlTqReq_Nm)
  If/5 -> Coordinate_MSA/Action
  [VVMC_MSAWhlTqReq_Nm] -> Coordinate_MSA/1(VVMC_MSAWhlTqReq_Nm)
  If/6 -> Coordinate_APS/Action
  [VTQD_DriverWhlTqDem_Nm] -> Coordinate_APS/1(VTQD_DriverWhlTqDem_Nm)
  If/7 -> Coordinate_DirverPedal/Action
  [VTQD_DriverWhlTqDem_Nm] -> Coordinate_DirverPedal/1(VTQD_DriverWhlTqDem_Nm)
  [VTQD_ADASForceIdle_enum] -> Merge5/7
  [VTQD_DriverWhlTqReq_Nm] -> Merge4/6
  [VTQD_MSAWhlTqReq_Nm] -> Merge4/4
  [VTQD_GearNoSuitReq_Nm] -> Merge4/1
  [VTQD_TqSourceCruz_enum] -> Merge5/3
  [VTQD_TqSourceInternal_enum] -> Merge5/6
  [VTQD_TqSourceMSA_enum] -> Merge5/4
  [VTQD_TqSourceAPS_enum] -> Merge5/5
  [VTQD_ADASForceIdleReq_Nm] -> Merge4/7
  Merge5/1 -> Data Type Conversion2/1
  [VTQD_TqSourceGearNoSuit_enum] -> Merge5/1
  Data Type Conversion2/1 -> VTQD_TqSource_enum/1  "VTQD_TqSource_enum"
  [VTQD_ADASWhlTqReq_Nm] -> Merge4/2
  [VTQD_APSWhlTqReq_Nm] -> Merge4/5
  [VTQD_CruzWhlTqReq_Nm] -> Merge4/3
  [VTQD_TqSourceADAS_enum] -> Merge5/2
  [VINP_HVBPwrAvailDchrg_kW] -> "Total Demand Capacity Torque "/1(VINP_HVBPwrAvailDchrg_kW)
  [VINP_HVBPwrAvailChrg_kW] -> "Total Demand Capacity Torque "/2(VINP_HVBPwrAvailChrg_kW)
  [VTQD_MotorLossTotal_kw] -> "Total Demand Capacity Torque "/3(VTQD_MotorLossTotal_kw)
  [VTQD_FrShaftSpd_rpm] -> "Total Demand Capacity Torque "/4(VTQD_FrShaftSpd_rpm)
  [VTQD_RrShaftSpd_rpm] -> "Total Demand Capacity Torque "/5(VTQD_RrShaftSpd_rpm)
  VTQD_RrShaftSpd_rpm/1 -> [VTQD_RrShaftSpd_rpm]
  VINP_HVBPwrAvailChrg_kW/1 -> [VINP_HVBPwrAvailChrg_kW]
  VINP_HVBPwrAvailDchrg_kW/1 -> [VINP_HVBPwrAvailDchrg_kW]
  VTQD_FrShaftSpd_rpm/1 -> [VTQD_FrShaftSpd_rpm]
  VTQD_MotorLossTotal_kw/1 -> [VTQD_MotorLossTotal_kw]
  "Total Demand Capacity Torque "/1(VTQD_TotalWhlTqCapMot_Nm) -> [VTQD_TotalWhlTqCapMot_Nm]
  "Total Demand Capacity Torque "/2(VTQD_TotalWhlTqCapGen_Nm) -> [VTQD_TotalWhlTqCapGen_Nm]
  Merge4/1 -> Saturation Dynamic/2, Switch/3
  [VTQD_TotalWhlTqCapMot_Nm] -> Saturation Dynamic/1
  [VTQD_TotalWhlTqCapGen_Nm] -> Saturation Dynamic/3
  Saturation Dynamic/1 -> Switch/1
  Switch/1 -> VTQD_CoordTqDem_Nm/1  "VTQD_CoordTqDem_Nm"
  Constant3/1 -> Switch/2
